simulink model "LAB_04_EX_1"  (R2022b)
settings: Solver=ode4  StartTime=0.0  StopTime=100  FixedStep=0.1  RelTol=1e-3
values from neighbouring files (symbols this model uses):
  A0 = eye(3,3)    [LAB_04.m]
  I = diag([0.07,0.055,0.025])    [LAB_04.m]
  q0 = [0;0;0;1]    [LAB_04.m]
  w0 = [0.45;0.52;0.55]    [LAB_04.m]
libraries: sharedutil x4, matrix_library x1
settings Model: Creator=ludov  LastModifiedBy=ludov

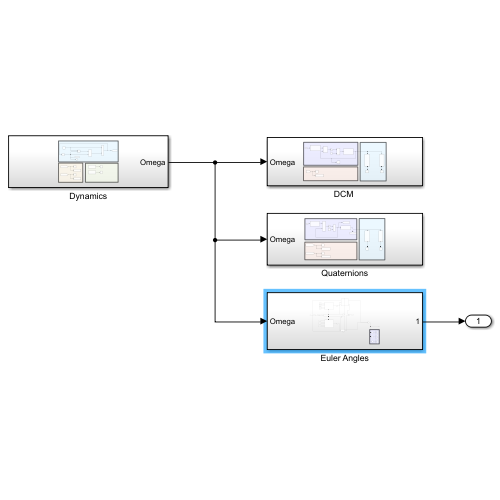
[thumbnail: Simulink's stored preview of the top-level diagram]
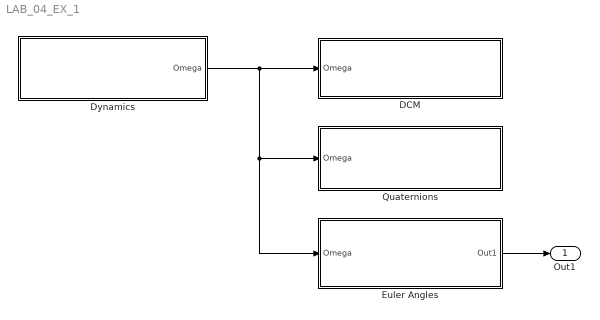
== system LAB_04_EX_1 ==
  "DCM " : Subsystem
  Dynamics : Subsystem
  Euler Angles : Subsystem
  Quaternions : Subsystem
  Out1 : Outport
  wires:
  Dynamics/1(Omega) -> Euler Angles/1(Omega), Quaternions/1(Omega), "DCM "/1(Omega)
  Euler Angles/1(Out1) -> Out1/1

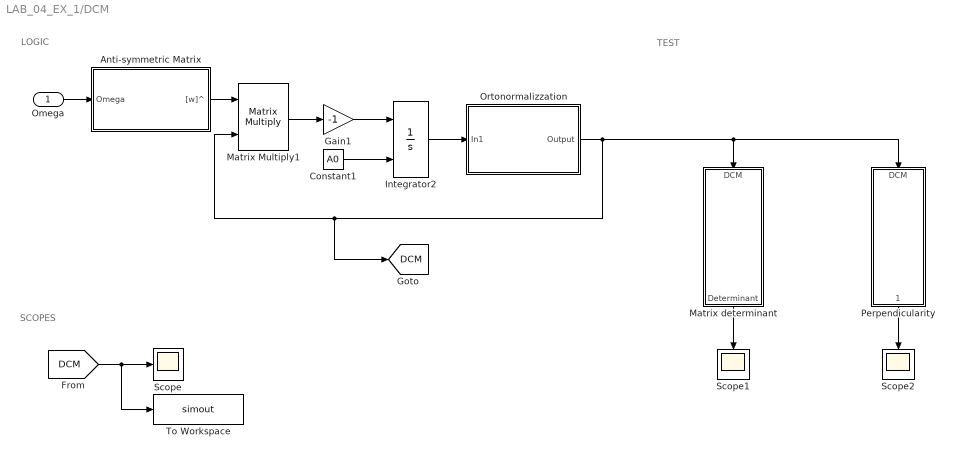
== system LAB_04_EX_1/DCM  ==
  note: SCOPES
  note: LOGIC
  note: TEST
  Omega : Inport
  Anti-symmetric Matrix : Subsystem
  Constant1 : Constant  Value=A0
  Gain1 : Gain  Gain=-1
  Integrator2 : Integrator  InitialConditionSource=external
  Matrix Multiply1 : Product  Multiplication=Matrix(*)
  Matrix determinant : Subsystem
  Ortonormalizzation : Subsystem
  Perpendicularity : Subsystem
  Scope : Scope
  Scope1 : Scope
  Scope2 : Scope
  To Workspace : ToWorkspace  VariableName=simout  SaveFormat=Timeseries  SampleTime=-1
  tag scope: DCM=global
  wires:
  [DCM] -> To Workspace/1, Scope/1
  Anti-symmetric Matrix/1("[w]^") -> Matrix Multiply1/1
  Integrator2/1 -> Ortonormalizzation/1(In1)
  Matrix Multiply1/1 -> Gain1/1
  Ortonormalizzation/1(Output) -> Perpendicularity/1(DCM), Matrix determinant/1(DCM), Matrix Multiply1/2, [DCM]
  Omega/1 -> Anti-symmetric Matrix/1(Omega)
  Gain1/1 -> Integrator2/1
  Constant1/1 -> Integrator2/2
  Matrix determinant/1(Determinant) -> Scope1/1
  Perpendicularity/1(Perpendicularity flag) -> Scope2/1

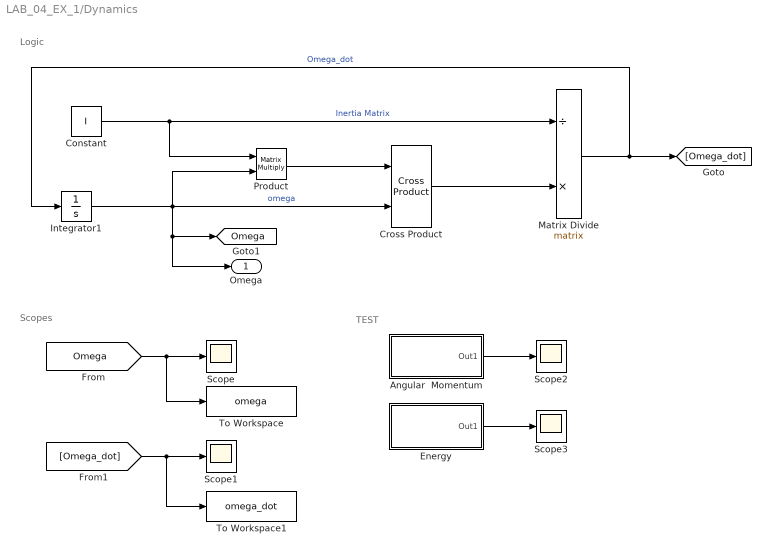
== system LAB_04_EX_1/Dynamics ==
  note: TEST
  note: Logic
  note: Scopes
  Angular  Momentum : Subsystem
  Constant : Constant  Value=I
  Cross Product : matrix_library/Cross Product
  Energy : Subsystem
  Integrator1 : Integrator  InitialCondition=w0
  Matrix Divide : Product  Inputs=/*  Multiplication=Matrix(*)
  Product : Product  Multiplication=Matrix(*)
  Scope{,1..3} (4 alike) : Scope
  To Workspace : ToWorkspace  VariableName=omega  SaveFormat=Timeseries  SampleTime=-1
  To Workspace1 : ToWorkspace  VariableName=omega_dot  SaveFormat=Timeseries  SampleTime=-1
  Omega : Outport
  tag scope: Omega=global
  wires:
  Product/1 -> Cross Product/1
  Integrator1/1 -> Cross Product/2, Product/2, Omega/1, [Omega]  "omega"
  Matrix Divide/1 -> [Omega_dot], Integrator1/1  "Omega_dot"
  Constant/1 -> Product/1, Matrix Divide/1  "Inertia Matrix"
  Cross Product/1 -> Matrix Divide/2
  [Omega] -> To Workspace/1, Scope/1
  [Omega_dot] -> To Workspace1/1, Scope1/1
  Angular  Momentum/1(Out1) -> Scope2/1
  Energy/1(Out1) -> Scope3/1

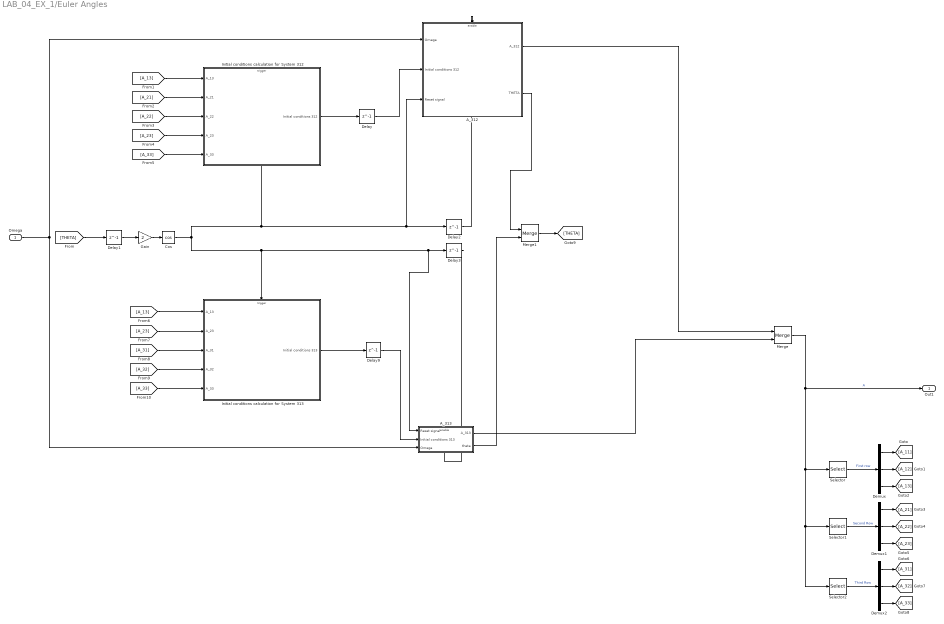
== system LAB_04_EX_1/Euler Angles ==
  Omega : Inport
  A_312 : Subsystem
  A_313 : Subsystem
  Cos : Trigonometry  Operator=cos
  Delay : Delay  DelayLength=1  InitialCondition=[0.1;0.1;0.1]
  Delay{1..3,9} (4 alike) : Delay  DelayLength=1
  Demux : Demux  Outputs=3
  Demux1 : Demux  Outputs=3
  Demux2 : Demux  Outputs=3
  Gain : Gain  Gain=2
  Initial conditions calculation for System 312 : Subsystem  TreatAsAtomicUnit=on
  Initial conditions calculation for System 313 : Subsystem  TreatAsAtomicUnit=on
  Merge : Merge
  Merge1 : Merge
  Selector : Selector  NumberOfDimensions=2  InputPortWidth=3  IndexOptions=Index vector (dialog),Index vector (dialog)  Indices=[1 2 3],1  OutputSizes=1,1
  Selector1 : Selector  NumberOfDimensions=2  InputPortWidth=3  IndexOptions=Index vector (dialog),Index vector (dialog)  Indices=[1 2 3],2  OutputSizes=1,1
  Selector2 : Selector  NumberOfDimensions=2  InputPortWidth=3  IndexOptions=Index vector (dialog),Index vector (dialog)  Indices=[1 2 3],3  OutputSizes=1,1
  Out1 : Outport
  wires:
  Demux1/3 -> [A_23]
  Merge/1 -> Selector1/1, Selector2/1, Selector/1, Out1/1  "A"
  Demux/1 -> [A_11]
  Demux1/1 -> [A_21]
  Selector1/1 -> Demux1/1  "Second Row"
  Demux/3 -> [A_13]
  Demux1/2 -> [A_22]
  Selector2/1 -> Demux2/1  "Third Row"
  A_313/1(A_313) -> Merge/2
  Merge1/1 -> [THETA]
  Demux2/2 -> [A_32]
  Demux/2 -> [A_12]
  A_312/1(A_312) -> Merge/1
  Selector/1 -> Demux/1  "First row"
  A_313/2(theta) -> Merge1/2
  Omega/1 -> A_312/1(Omega), A_313/3(Omega)
  Demux2/3 -> [A_33]
  Demux2/1 -> [A_31]
  A_312/2(THETA) -> Merge1/1
  Delay9/1 -> A_313/2(Initial conditions 313)
  [A_23] -> Initial conditions calculation for System 313/2(A_23)
  [A_32] -> Initial conditions calculation for System 313/4(A_32)
  [A_22] -> Initial conditions calculation for System 312/3(A_22)
  [A_13] -> Initial conditions calculation for System 313/1(A_13)
  Initial conditions calculation for System 313/1(Initial conditions 313) -> Delay9/1
  [A_33] -> Initial conditions calculation for System 313/5(A_33)
  [A_31] -> Initial conditions calculation for System 313/3(A_31)
  [A_23] -> Initial conditions calculation for System 312/4(A_23)
  Delay1/1 -> Gain/1
  Gain/1 -> Cos/1
  Initial conditions calculation for System 312/1(Initial conditions 312) -> Delay/1
  [THETA] -> Delay1/1
  [A_13] -> Initial conditions calculation for System 312/1(A_13)
  [A_21] -> Initial conditions calculation for System 312/2(A_21)
  [A_33] -> Initial conditions calculation for System 312/5(A_33)
  Delay/1 -> A_312/2(Initial conditions 312)
  Delay2/1 -> A_312/Enable
  Delay3/1 -> A_313/Enable
  Cos/1 -> Delay2/1, A_312/3(Reset signal), Initial conditions calculation for System 312/Trigger, Initial conditions calculation for System 313/Trigger, A_313/1(Reset signal), Delay3/1

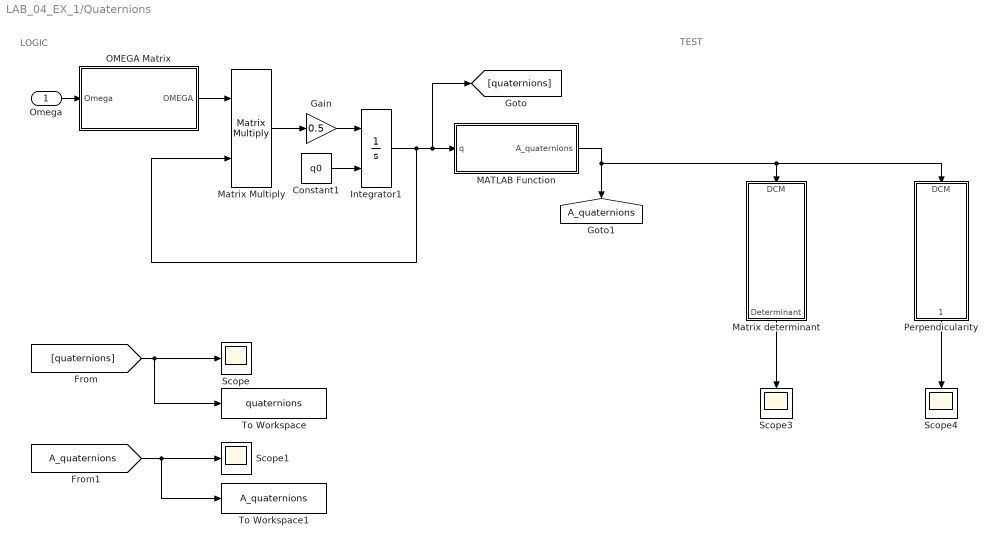
== system LAB_04_EX_1/Quaternions ==
  note: LOGIC
  note: TEST
  Omega : Inport
  Constant1 : Constant  Value=q0
  Gain : Gain  Gain=0.5
  Integrator1 : Integrator  InitialConditionSource=external  InitialCondition=q0
  MATLAB Function : MATLAB Function  TreatAsAtomicUnit=on
  Matrix Multiply : Product  Multiplication=Matrix(*)
  Matrix determinant : Subsystem
  OMEGA Matrix : Subsystem
  Perpendicularity : Subsystem
  Scope{,1,3..4} (4 alike) : Scope
  To Workspace : ToWorkspace  VariableName=quaternions  SaveFormat=Timeseries  SampleTime=-1
  To Workspace1 : ToWorkspace  VariableName=A_quaternions  SaveFormat=Timeseries  SampleTime=-1
  tag scope: A_quaternions=global
  wires:
  Omega/1 -> OMEGA Matrix/1(Omega)
  OMEGA Matrix/1(OMEGA) -> Matrix Multiply/1
  [quaternions] -> Scope/1, To Workspace/1
  [A_quaternions] -> To Workspace1/1, Scope1/1
  MATLAB Function/1(A_quaternions) -> [A_quaternions], Perpendicularity/1(DCM), Matrix determinant/1(DCM)
  Matrix Multiply/1 -> Gain/1
  Matrix determinant/1(Determinant) -> Scope3/1
  Perpendicularity/1(Perpendicularity flag) -> Scope4/1
  Gain/1 -> Integrator1/1
  Integrator1/1 -> Matrix Multiply/2, [quaternions], MATLAB Function/1(q)
  Constant1/1 -> Integrator1/2

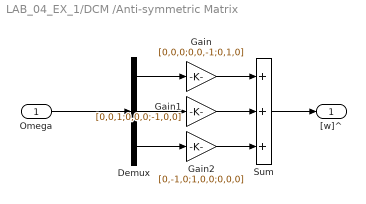
== system LAB_04_EX_1/DCM /Anti-symmetric Matrix ==
  Omega : Inport
  Demux : Demux  Outputs=3
  Gain : Gain  Gain=[0,0,0;0,0,-1;0,1,0]
  Gain1 : Gain  Gain=[0,0,1;0,0,0;-1,0,0]
  Gain2 : Gain  Gain=[0,-1,0;1,0,0;0,0,0]
  Sum : Sum  Inputs=+++
  "[w]^" : Outport
  wires:
  Sum/1 -> "[w]^"/1
  Demux/1 -> Gain/1
  Gain/1 -> Sum/1
  Demux/3 -> Gain2/1
  Gain2/1 -> Sum/3
  Demux/2 -> Gain1/1
  Gain1/1 -> Sum/2
  Omega/1 -> Demux/1

== system LAB_04_EX_1/DCM /Matrix determinant ==
  DCM : Inport
  Determinant of 3x3 Matrix : sharedutil/Determinant of 3x3 Matrix  aMode=aMode
      settings: LibrarySourceBlock=|
      | aerolibutil/Determinant of
      | 3x3 Matrix
  Determinant : Outport
  wires:
  Determinant of 3x3 Matrix/1 -> Determinant/1
  DCM/1 -> Determinant of 3x3 Matrix/1

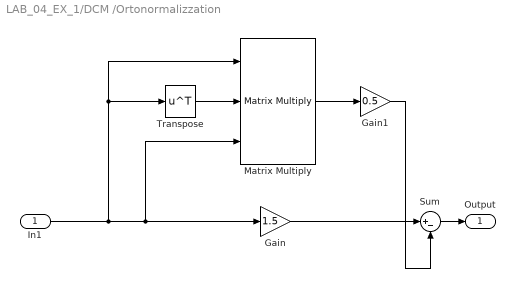
== system LAB_04_EX_1/DCM /Ortonormalizzation ==
  In1 : Inport
  Gain : Gain  Gain=1.5
  Gain1 : Gain  Gain=0.5
  Matrix Multiply : Product  Inputs=3  Multiplication=Matrix(*)
  Sum : Sum  Inputs=|+-
  Transpose : Math  Operator=transpose
  Output : Outport
  wires:
  Matrix Multiply/1 -> Gain1/1
  Gain/1 -> Sum/1
  In1/1 -> Matrix Multiply/3, Gain/1, Transpose/1, Matrix Multiply/1
  Gain1/1 -> Sum/2
  Transpose/1 -> Matrix Multiply/2
  Sum/1 -> Output/1

== system LAB_04_EX_1/DCM /Perpendicularity ==
  DCM : Inport
  MATLAB Function2 : MATLAB Function  TreatAsAtomicUnit=on
  Perpendicularity flag : Outport
  wires:
  MATLAB Function2/1(perpendicularity_flag) -> Perpendicularity flag/1
  DCM/1 -> MATLAB Function2/1(DCM)

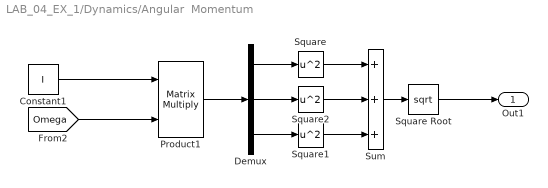
== system LAB_04_EX_1/Dynamics/Angular  Momentum ==
  Constant1 : Constant  Value=I
  Demux : Demux  Outputs=3
  Product1 : Product  Multiplication=Matrix(*)
  Square : Math  Operator=square
  Square Root : Sqrt
  Square1 : Math  Operator=square
  Square2 : Math  Operator=square
  Sum : Sum  Inputs=+++
  Out1 : Outport
  wires:
  [Omega] -> Product1/2
  Constant1/1 -> Product1/1
  Product1/1 -> Demux/1
  Square Root/1 -> Out1/1
  Demux/1 -> Square/1
  Demux/2 -> Square2/1
  Demux/3 -> Square1/1
  Square/1 -> Sum/1
  Square2/1 -> Sum/2
  Square1/1 -> Sum/3
  Sum/1 -> Square Root/1

== system LAB_04_EX_1/Dynamics/Energy ==
  Constant1 : Constant  Value=I
  Gain : Gain  Gain=0.5
  Matrix Multiply : Product  Multiplication=Matrix(*)
  Matrix Multiply1 : Product  Multiplication=Matrix(*)
  Transpose : Math  Operator=transpose
  Out1 : Outport
  wires:
  Matrix Multiply1/1 -> Gain/1
  Matrix Multiply/1 -> Matrix Multiply1/1
  [Omega] -> Matrix Multiply1/2, Transpose/1
  Transpose/1 -> Matrix Multiply/1
  Gain/1 -> Out1/1
  Constant1/1 -> Matrix Multiply/2

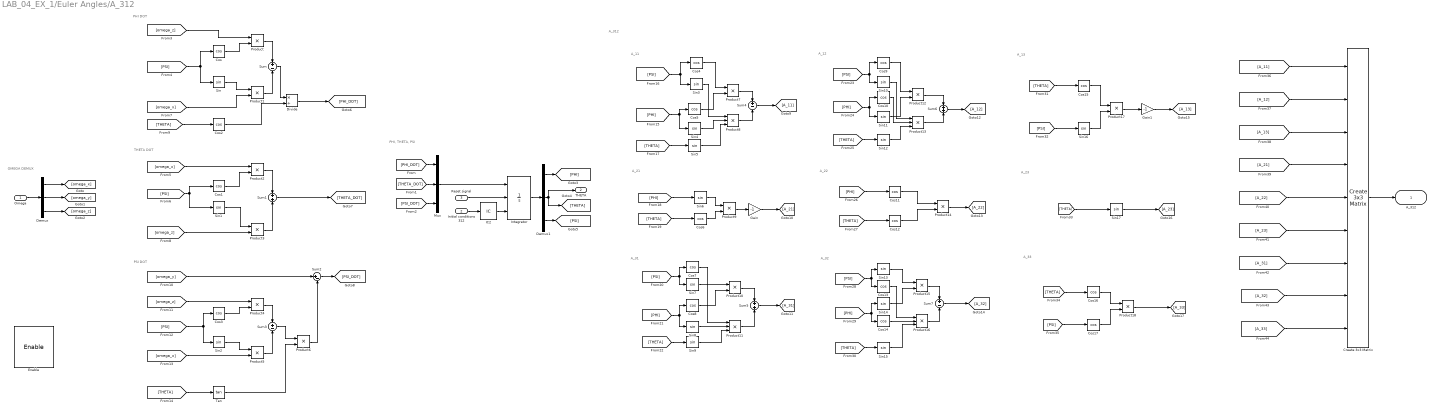
== system LAB_04_EX_1/Euler Angles/A_312 ==
  note: PHI, THETA, PSI
  note: OMEGA DEMUX
  note: PHI DOT
  note: PSI DOT
  note: THETA DOT
  note: A_31
  note: A_23
  note: A_33
  note: A_32
  note: A_312
  note: A_22
  note: A_12
  note: A_21
  note: A_13
  note: A_11
  Omega : Inport
  Initial conditions 312 : Inport  Port=2
  Reset signal : Inport  Port=3
  Enable : EnablePort
  Cos{,1..17} (18 alike) : Trigonometry  Operator=cos
  Create 3x3 Matrix : sharedutil/Create 3x3 Matrix  aMode=aMode
      settings: LibrarySourceBlock=aerolibutil/Create 3x3 Matrix
  Demux : Demux  Outputs=3
  Demux1 : Demux  Outputs=3
  Divide : Product  Inputs=*/
  Gain : Gain  Gain=-1
  Gain1 : Gain  Gain=-1
  IC2 : InitialCondition  Value=[0;0;0]
  Integrator : Integrator  ExternalReset=rising  InitialConditionSource=external
  Mux : Mux  Inputs=3
  Product{,1..7,9..10,12,14..15,17..18} (15 alike) : Product
  Product{8,11,13,16} (4 alike) : Product  Inputs=3
  Sin{,1..17} (18 alike) : Trigonometry
  Sum{,3..4,7} (4 alike) : Sum  Inputs=+-
  Sum1 : Sum
  Sum2 : Sum  Inputs=|+-
  Sum5 : Sum
  Sum6 : Sum
  Tan : Trigonometry  Operator=tan
  A_312 : Outport
  THETA : Outport  Port=2
  wires:
  Omega/1 -> Demux/1
  Demux/1 -> [omega_x]
  Demux/2 -> [omega_y]
  Demux/3 -> [omega_z]
  [omega_x] -> Product1/2
  [PSI] -> Sin/1, Cos/1
  [omega_x] -> Product2/1
  [THETA] -> Cos2/1
  Sin/1 -> Product1/1
  Sin2/1 -> Product5/1
  Cos3/1 -> Product4/2
  Tan/1 -> Product6/2
  Divide/1 -> [PHI_DOT]
  Product4/1 -> Sum3/1
  Sum1/1 -> [THETA_DOT]
  Product/1 -> Sum/1
  Sum/1 -> Divide/1
  Cos/1 -> Product/2
  [omega_x] -> Product5/2
  Cos2/1 -> Divide/2
  Product3/1 -> Sum1/2
  [omega_y] -> Sum2/1
  Sum2/1 -> [PSI_DOT]
  Sum3/1 -> Product6/1
  [THETA] -> Tan/1
  Product2/1 -> Sum1/1
  [PSI] -> Sin2/1, Cos3/1
  [PSI] -> Sin1/1, Cos1/1
  Product5/1 -> Sum3/2
  Cos1/1 -> Product2/2
  Sin1/1 -> Product3/1
  Product1/1 -> Sum/2
  [omega_z] -> Product4/1
  Product6/1 -> Sum2/2
  [omega_z] -> Product3/2
  [omega_z] -> Product/1
  [PHI] -> Cos11/1
  [A_21] -> Create 3x3 Matrix/4
  Sin3/1 -> Product8/1
  [A_31] -> Create 3x3 Matrix/7
  [A_32] -> Create 3x3 Matrix/8
  Product17/1 -> Gain1/1
  [A_22] -> Create 3x3 Matrix/5
  [A_23] -> Create 3x3 Matrix/6
  [A_13] -> Create 3x3 Matrix/3
  [THETA] -> Cos6/1
  [A_12] -> Create 3x3 Matrix/2
  Sin12/1 -> Product13/3
  Sum7/1 -> [A_32]
  [A_11] -> Create 3x3 Matrix/1
  [PHI] -> Sin11/1, Cos10/1
  Create 3x3 Matrix/1 -> A_312/1
  Cos17/1 -> Product18/2
  [THETA] -> Sin12/1
  Product15/1 -> Sum7/1
  Sin9/1 -> Product11/3
  Sin16/1 -> Product17/2
  Product18/1 -> [A_33]
  Cos6/1 -> Product9/2
  Gain1/1 -> [A_13]
  [THETA] -> Sin17/1
  Cos15/1 -> Product17/1
  [PSI] -> Cos17/1
  Product8/1 -> Sum4/2
  Cos16/1 -> Product18/1
  [PHI] -> Sin14/1, Cos14/1
  [THETA] -> Cos16/1
  [THETA] -> Cos15/1
  Sin11/1 -> Product12/2
  Cos14/1 -> Product16/2
  Sum6/1 -> [A_12]
  Sin15/1 -> Product16/3
  [PSI] -> Sin10/1, Cos9/1
  Cos8/1 -> Product10/2
  Cos12/1 -> Product14/2
  Cos11/1 -> Product14/1
  Product16/1 -> Sum7/2
  Cos7/1 -> Product11/1
  [THETA] -> Cos12/1
  [PSI] -> Cos13/1, Sin13/1
  Product14/1 -> [A_22]
  Sin8/1 -> Product11/2
  [THETA] -> Sin15/1
  Cos9/1 -> Product12/1
  Sum4/1 -> [A_11]
  Sin13/1 -> Product15/1
  Gain/1 -> [A_21]
  [PHI] -> Sin6/1
  Sum5/1 -> [A_31]
  Sin14/1 -> Product15/2
  Product10/1 -> Sum5/1
  Product9/1 -> Gain/1
  Cos10/1 -> Product13/2
  Cos13/1 -> Product16/1
  Sin10/1 -> Product13/1
  [PSI] -> Sin3/1, Cos4/1
  [THETA] -> Sin9/1
  Sin6/1 -> Product9/1
  Product13/1 -> Sum6/2
  Product11/1 -> Sum5/2
  [THETA] -> Sin5/1
  Sin7/1 -> Product10/1
  [PHI] -> Cos8/1, Sin8/1
  Sin4/1 -> Product8/2
  [PSI] -> Sin16/1
  [A_33] -> Create 3x3 Matrix/9
  [PHI] -> Cos5/1, Sin4/1
  Sin17/1 -> [A_23]
  [PSI] -> Sin7/1, Cos7/1
  Sin5/1 -> Product8/3
  Cos5/1 -> Product7/2
  Product12/1 -> Sum6/1
  Product7/1 -> Sum4/1
  Cos4/1 -> Product7/1
  Mux/1 -> Integrator/1
  [PSI_DOT] -> Mux/3
  Initial conditions 312/1 -> IC2/1
  IC2/1 -> Integrator/3
  Demux1/3 -> [PSI]
  Reset signal/1 -> Integrator/2
  Demux1/2 -> THETA/1, [THETA]
  Demux1/1 -> [PHI]
  [PHI_DOT] -> Mux/1
  Integrator/1 -> Demux1/1
  [THETA_DOT] -> Mux/2

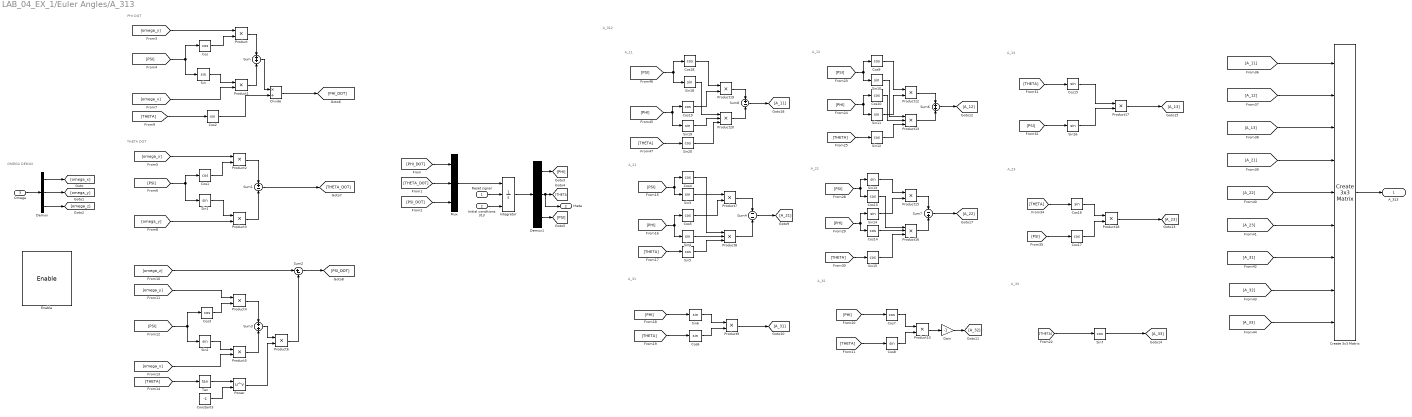
== system LAB_04_EX_1/Euler Angles/A_313 ==
  note: OMEGA DEMUX
  note: A_312
  note: THETA DOT
  note: PHI DOT
  note: A_11
  note: A_12
  note: A_13
  note: A_21
  note: A_31
  note: A_32
  note: A_33
  note: A_22
  note: A_23
  Reset signal : Inport
  Initial conditions 313 : Inport  Port=2
  Omega : Inport  Port=3
  Enable : EnablePort
  Constant3 : Constant  Value=-1
  Cos{,1,3..5,7,9..10,13..14,17..19} (13 alike) : Trigonometry  Operator=cos
  Cos{2,6,8,15..16} (5 alike) : Trigonometry
  Create 3x3 Matrix : sharedutil/Create 3x3 Matrix  aMode=aMode
      settings: LibrarySourceBlock=aerolibutil/Create 3x3 Matrix
  Demux : Demux  Outputs=3
  Demux1 : Demux  Outputs=3
  Divide : Product  Inputs=*/
  Gain : Gain  Gain=-1
  Integrator : Integrator  ExternalReset=falling  InitialConditionSource=external
  Mux : Mux  Inputs=3
  Power : Math  Operator=pow
  Product{,1..7,9..10,12,15,17..19} (15 alike) : Product
  Product{8,13,16,20} (4 alike) : Product  Inputs=3
  Sin{,1..4,6,10..11,13..14,16,18..19} (13 alike) : Trigonometry
  Sin{5,7,12,15,20} (5 alike) : Trigonometry  Operator=cos
  Sum : Sum
  Sum1 : Sum  Inputs=+-
  Sum2 : Sum  Inputs=|+-
  Sum3 : Sum
  Sum4 : Sum  Inputs=--
  Sum6 : Sum
  Sum7 : Sum  Inputs=-+
  Sum8 : Sum  Inputs=+-
  Tan : Trigonometry  Operator=tan
  A_313 : Outport
  theta : Outport  Port=2
  wires:
  Omega/1 -> Demux/1
  Demux/1 -> [omega_x]
  Demux/2 -> [omega_y]
  Demux/3 -> [omega_z]
  [A_21] -> Create 3x3 Matrix/4
  [A_31] -> Create 3x3 Matrix/7
  [A_32] -> Create 3x3 Matrix/8
  [A_22] -> Create 3x3 Matrix/5
  [A_23] -> Create 3x3 Matrix/6
  [A_13] -> Create 3x3 Matrix/3
  [A_12] -> Create 3x3 Matrix/2
  [A_11] -> Create 3x3 Matrix/1
  Create 3x3 Matrix/1 -> A_313/1
  [A_33] -> Create 3x3 Matrix/9
  Power/1 -> Product6/2
  Tan/1 -> Power/1
  [omega_x] -> Product1/2
  Cos1/1 -> Product2/2
  [THETA] -> Cos2/1
  Constant3/1 -> Power/2
  [omega_y] -> Product3/2
  Divide/1 -> [PHI_DOT]
  [omega_x] -> Product5/2
  [THETA] -> Tan/1
  Cos/1 -> Product/2
  Sin/1 -> Product1/1
  Sin1/1 -> Product3/1
  [PSI] -> Sin1/1, Cos1/1
  Cos2/1 -> Divide/2
  Product1/1 -> Sum/2
  Sum/1 -> Divide/1
  Product3/1 -> Sum1/2
  Sum1/1 -> [THETA_DOT]
  [omega_y] -> Product/1
  [PSI] -> Sin2/1, Cos3/1
  Product6/1 -> Sum2/2
  Product2/1 -> Sum1/1
  Product5/1 -> Sum3/2
  Sum2/1 -> [PSI_DOT]
  Product/1 -> Sum/1
  Sin2/1 -> Product5/1
  Sum3/1 -> Product6/1
  [omega_x] -> Product2/1
  [omega_z] -> Sum2/1
  [omega_y] -> Product4/1
  Product4/1 -> Sum3/1
  [PSI] -> Sin/1, Cos/1
  Cos3/1 -> Product4/2
  Sum8/1 -> [A_11]
  [PSI] -> Sin18/1, Cos18/1
  Cos19/1 -> Product19/2
  Sin20/1 -> Product20/3
  Product20/1 -> Sum8/2
  [PHI] -> Cos19/1, Sin19/1
  Product19/1 -> Sum8/1
  [THETA] -> Sin20/1
  Cos18/1 -> Product19/1
  Sin18/1 -> Product20/1
  Sin19/1 -> Product20/2
  Sum6/1 -> [A_12]
  Sin10/1 -> Product13/1
  Sin12/1 -> Product13/3
  Cos9/1 -> Product12/1
  [THETA] -> Sin12/1
  Cos10/1 -> Product13/2
  Product13/1 -> Sum6/2
  [PSI] -> Sin10/1, Cos9/1
  [PHI] -> Sin11/1, Cos10/1
  Product12/1 -> Sum6/1
  Sin11/1 -> Product12/2
  Cos15/1 -> Product17/1
  [THETA] -> Cos15/1
  Sin16/1 -> Product17/2
  [PSI] -> Sin16/1
  Product17/1 -> [A_13]
  [THETA] -> Sin5/1
  [PHI] -> Cos5/1, Sin4/1
  Sum4/1 -> [A_21]
  Cos4/1 -> Product8/1
  Sin4/1 -> Product8/2
  Sin5/1 -> Product8/3
  Sin3/1 -> Product7/1
  Cos5/1 -> Product7/2
  Product8/1 -> Sum4/2
  Product7/1 -> Sum4/1
  [PSI] -> Sin3/1, Cos4/1
  [THETA] -> Cos6/1
  Product9/1 -> [A_31]
  [PHI] -> Sin6/1
  Sin6/1 -> Product9/1
  Cos6/1 -> Product9/2
  Gain/1 -> [A_32]
  [PHI] -> Cos7/1
  Product10/1 -> Gain/1
  Cos7/1 -> Product10/1
  Cos8/1 -> Product10/2
  [THETA] -> Cos8/1
  [THETA] -> Sin7/1
  Sin7/1 -> [A_33]
  Cos14/1 -> Product16/2
  Sin13/1 -> Product15/1
  Sin14/1 -> Product15/2
  [THETA] -> Sin15/1
  Cos13/1 -> Product16/1
  Sum7/1 -> [A_22]
  Product16/1 -> Sum7/2
  Sin15/1 -> Product16/3
  [PSI] -> Cos13/1, Sin13/1
  Product15/1 -> Sum7/1
  [PHI] -> Sin14/1, Cos14/1
  Cos16/1 -> Product18/1
  Cos17/1 -> Product18/2
  Product18/1 -> [A_23]
  [PSI] -> Cos17/1
  [THETA] -> Cos16/1
  Demux1/1 -> [PHI]
  [PSI_DOT] -> Mux/3
  [THETA_DOT] -> Mux/2
  Initial conditions 313/1 -> Integrator/3
  Reset signal/1 -> Integrator/2
  Demux1/2 -> theta/1, [THETA]
  Demux1/3 -> [PSI]
  Mux/1 -> Integrator/1
  [PHI_DOT] -> Mux/1
  Integrator/1 -> Demux1/1

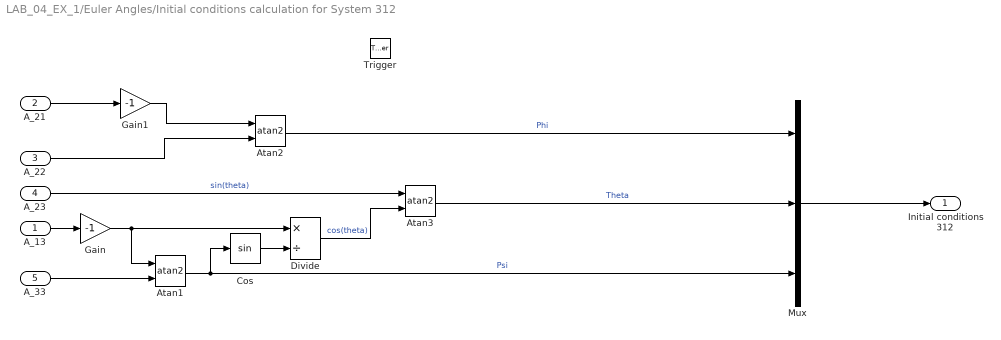
== system LAB_04_EX_1/Euler Angles/Initial conditions calculation for System 312 ==
  A_13 : Inport
  A_21 : Inport  Port=2
  A_22 : Inport  Port=3
  A_23 : Inport  Port=4
  A_33 : Inport  Port=5
  Trigger : TriggerPort  VariantControl=(inherit)
  Atan1 : Trigonometry  Operator=atan2
  Atan2 : Trigonometry  Operator=atan2
  Atan3 : Trigonometry  Operator=atan2
  Cos : Trigonometry
  Divide : Product  Inputs=*/
  Gain : Gain  Gain=-1
  Gain1 : Gain  Gain=-1
  Mux : Mux  Inputs=3
  Initial conditions 312 : Outport  InitialOutput=[0;0;0]
  wires:
  Mux/1 -> Initial conditions 312/1
  A_21/1 -> Gain1/1
  A_22/1 -> Atan2/2
  Atan2/1 -> Mux/1  "Phi"
  Atan1/1 -> Cos/1, Mux/3  "Psi"
  Cos/1 -> Divide/2
  Divide/1 -> Atan3/2  "cos(theta)"
  A_23/1 -> Atan3/1  "sin(theta)"
  Atan3/1 -> Mux/2  "Theta"
  Gain1/1 -> Atan2/1
  A_33/1 -> Atan1/2
  A_13/1 -> Gain/1
  Gain/1 -> Atan1/1, Divide/1

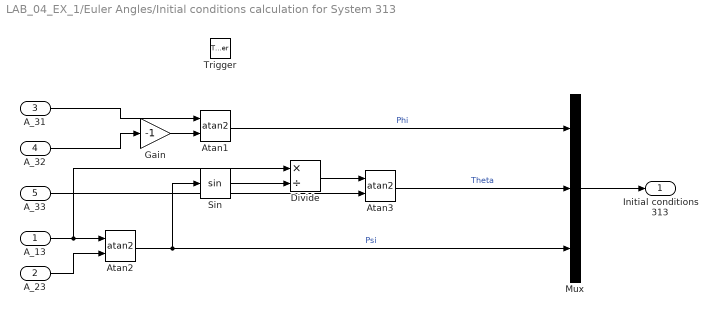
== system LAB_04_EX_1/Euler Angles/Initial conditions calculation for System 313 ==
  A_13 : Inport
  A_23 : Inport  Port=2
  A_31 : Inport  Port=3
  A_32 : Inport  Port=4
  A_33 : Inport  Port=5
  Trigger : TriggerPort  TriggerType=falling  VariantControl=(inherit)
  Atan1 : Trigonometry  Operator=atan2
  Atan2 : Trigonometry  Operator=atan2
  Atan3 : Trigonometry  Operator=atan2
  Divide : Product  Inputs=*/
  Gain : Gain  Gain=-1
  Mux : Mux  Inputs=3
  Sin : Trigonometry
  Initial conditions 313 : Outport
  wires:
  Mux/1 -> Initial conditions 313/1
  A_13/1 -> Divide/1, Atan2/1
  A_23/1 -> Atan2/2
  Atan2/1 -> Sin/1, Mux/3  "Psi"
  A_31/1 -> Atan1/1
  A_32/1 -> Gain/1
  Atan3/1 -> Mux/2  "Theta"
  A_33/1 -> Atan3/2
  Divide/1 -> Atan3/1
  Sin/1 -> Divide/2
  Atan1/1 -> Mux/1  "Phi"
  Gain/1 -> Atan1/2

== system LAB_04_EX_1/Quaternions/Matrix determinant ==
  DCM : Inport
  Determinant of 3x3 Matrix : sharedutil/Determinant of 3x3 Matrix  aMode=aMode
      settings: LibrarySourceBlock=|
      | aerolibutil/Determinant of
      | 3x3 Matrix
  Determinant : Outport
  wires:
  Determinant of 3x3 Matrix/1 -> Determinant/1
  DCM/1 -> Determinant of 3x3 Matrix/1

== system LAB_04_EX_1/Quaternions/OMEGA Matrix ==
  Omega : Inport
  Demux : Demux  Outputs=3
  Gain : Gain  Gain=[0 0 0 1; 0 0 1 0; 0 -1 0 0; -1 0 0 0]
  Gain1 : Gain  Gain=[0 0 -1 0; 0 0 0 1; 1 0 0 0; 0 -1 0 0]
  Gain2 : Gain  Gain=[0 1 0 0; -1 0 0 0; 0 0 0 1; 0 0 -1 0]
  Sum : Sum  Inputs=+++
  OMEGA : Outport
  wires:
  Sum/1 -> OMEGA/1
  Demux/1 -> Gain/1
  Gain/1 -> Sum/1
  Demux/3 -> Gain2/1
  Gain2/1 -> Sum/3
  Demux/2 -> Gain1/1
  Gain1/1 -> Sum/2
  Omega/1 -> Demux/1

== system LAB_04_EX_1/Quaternions/Perpendicularity ==
  DCM : Inport
  MATLAB Function2 : MATLAB Function  TreatAsAtomicUnit=on
  Perpendicularity flag : Outport
  wires:
  MATLAB Function2/1(perpendicularity_flag) -> Perpendicularity flag/1
  DCM/1 -> MATLAB Function2/1(DCM)

== matlab function LAB_04_EX_1/Quaternions/MATLAB Function ==
  data: q input; A_quaternions output
function A_quaternions = fcn_quaternions(q)

% Define the elements
    q1 = q(1);
    q2 = q(2);
    q3 = q(3);
    q4 = q(4);

% Calculate the DCM

    A_quaternions =     [   q1^2 - q2^2 - q3^2 + q4^2   ,   2*(q1*q2 + q3*q4)           ,   2*(q1*q3 - q2*q4);
                            2*(q1*q2 - q3*q4)           ,   -q1^2 + q2^2 - q3^2 + q4^2  ,   2*(q2*q3 + q1*q4);
                            2*(q1*q3 + q2*q4)           ,   2*(q3*q2 - q1*q4)           ,   -q1^2 - q2^2 + q3^2 + q4^2];

end

== matlab function LAB_04_EX_1/DCM /Perpendicularity/MATLAB Function2 ==
  data: DCM input; perpendicularity_flag output
function perpendicularity_flag = fcn(DCM)
    

perpendicularity_flag =zeros(3,1);

    x   = DCM(1,:);
    y   = DCM(2,:);
    z   = DCM(3,:);

    perpendicularity_flag(1)=dot(x,y);
    perpendicularity_flag(2)=dot(x,z);
    perpendicularity_flag(1)=dot(z,y);

end

== matlab function LAB_04_EX_1/Quaternions/Perpendicularity/MATLAB Function2 ==
  data: DCM input; perpendicularity_flag output
function perpendicularity_flag = fcn(DCM)
    

perpendicularity_flag =zeros(3,1);

    x   = DCM(1,:);
    y   = DCM(2,:);
    z   = DCM(3,:);

    perpendicularity_flag(1)=dot(x,y);
    perpendicularity_flag(2)=dot(x,z);
    perpendicularity_flag(1)=dot(z,y);

end
